simulink model "ACSEDC_motor"  (R2024a)
settings: Solver=VariableStepAuto  StartTime=0.0  StopTime=20  RelTol=1e-3
values from neighbouring files (symbols this model uses):
  B = 0.01    [SEDC_motor.m]
  KePhi = 1.6    [SEDC_motor.m]
  Ra = 0.5    [SEDC_motor.m]
  tau_a = La/Ra    [SEDC_motor.m]
  tau_m = J/B    (= 500)    [SEDC_motor.m]
  TL = 20    [SEDC_motor.m]
  Va = 200    [SEDC_motor.m]
settings Model: Creator=NADAAN  LastModifiedBy=NADAAN

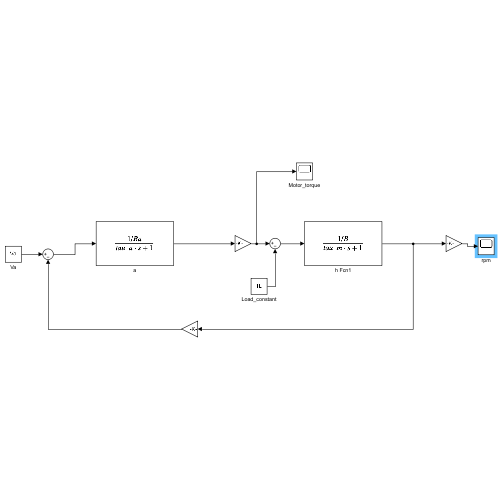
[thumbnail: Simulink's stored preview of the top-level diagram]
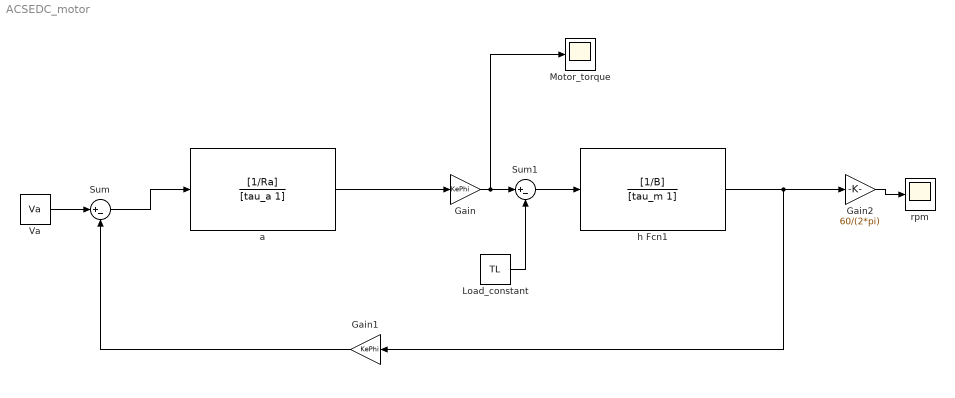
== system ACSEDC_motor ==
  Gain : Gain  Gain=KePhi
  Gain1 : Gain  Gain=KePhi
  Gain2 : Gain  Gain=60/(2*pi)
  Load_constant : Constant  Value=TL
  Motor_torque : Scope
  Sum : Sum  Inputs=|+-
  Sum1 : Sum  Inputs=|+-
  Va : Constant  Value=Va
  a : TransferFcn  Numerator=[1/Ra]  Denominator=[tau_a 1]  ContinuousStateAttributes="\"m1\""
  h Fcn1 : TransferFcn  Numerator=[1/B]  Denominator=[tau_m 1]  ContinuousStateAttributes="\"m2\""
  rpm : Scope
  wires:
  Va/1 -> Sum/1
  Sum/1 -> a/1
  a/1 -> Gain/1
  Gain/1 -> Motor_torque/1, Sum1/1
  Load_constant/1 -> Sum1/2
  Sum1/1 -> h Fcn1/1
  h Fcn1/1 -> Gain1/1, Gain2/1
  Gain1/1 -> Sum/2
  Gain2/1 -> rpm/1
